simulink model "ThreeDOF_Rocket_Simulator_CD"  (R2023b)
settings: Solver=VariableStepAuto  StartTime=0.0  StopTime=40  FixedStep=1e-4  RelTol=1e-6
libraries: shared3dof x1
settings Model: Creator=giuse  LastModifiedBy=aleco
settings SolverCC: EnableFixedStepZeroCrossing=on
settings DataIOCC: SaveState=on
settings DebuggingCC: UnconnectedInputMsg=warning  UnconnectedOutputMsg=warning  UnconnectedLineMsg=warning
settings ModelReferenceCC: EnableRefExpFcnMdlSchedulingChecks=on
settings RTWCC: DLArmComputeVersion=19.05

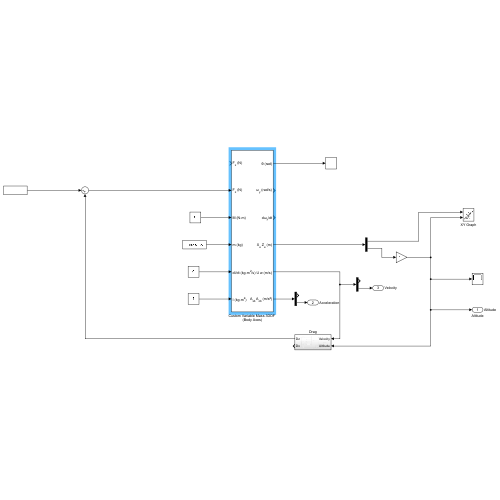
[thumbnail: Simulink's stored preview of the top-level diagram]
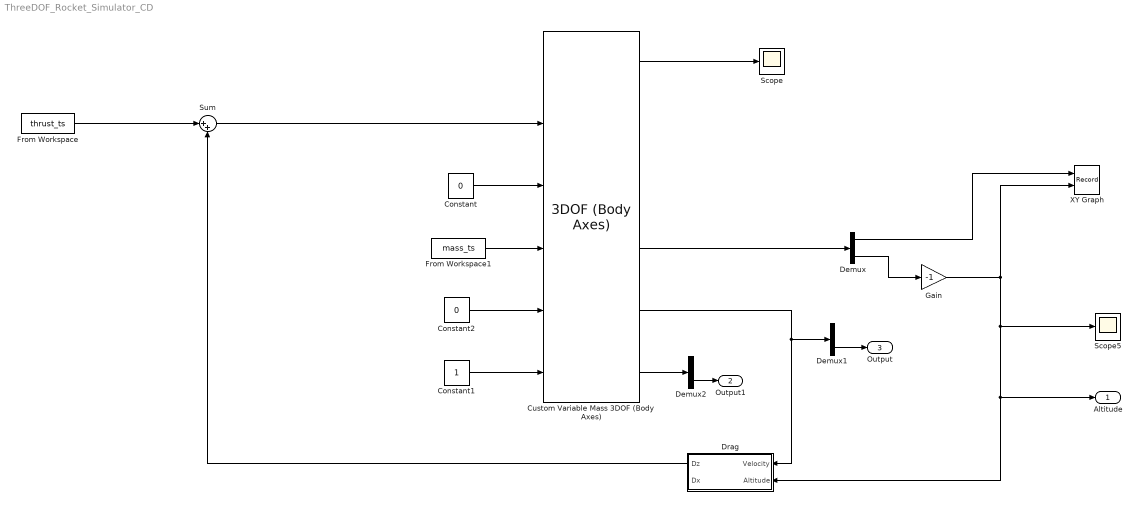
== system ThreeDOF_Rocket_Simulator_CD ==
  Constant : Constant  Value=0
  Constant1 : Constant
  Constant2 : Constant  Value=0
  Custom Variable Mass 3DOF (Body Axes) : shared3dof/3DOF (Body Axes)  units=Metric (MKS)  mtype=Custom Variable  v_ini=0  theta_ini=pi  alpha_ini=0  pos_ini=[0 0]  q_ini=0  mass=1.0  mass_e=0.5  mass_f=3.0  Iyy=1.0  Iyy_e=0.5  Iyy_f=3.0  g_in=Internal  g=9.81  vre_flag=off  abi_flag=off  aMode=0  vel_statename=''  theta_statename=''  pos_statename=''  q_statename=''  mass_statename=''
  Demux : Demux  Outputs=2
  Demux1 : Demux  Outputs=2
  Demux2 : Demux  Outputs=2
  Drag : Subsystem
  From Workspace : FromWorkspace  VariableName=thrust_ts
  From Workspace1 : FromWorkspace  VariableName=mass_ts
  Gain : Gain  Gain=-1
  Scope : Scope
  Scope5 : Scope
  Sum : Sum  Inputs=|++
  XY Graph : Record  FileSettingsInternal="{\"entries\":[{\"content\":{\"excelSettings\":{\"content\":{},\"type\":\"Streamout.ExcelSettings\"}},\"type\":\"Streamout.FileSettingStorage\",\"uuid\":\"\"}],\"packageUris\":[\"http:\\/\\/schema.mathworks.com\\/mf0\\/streamout_blocks\\/R2020a\"],\"version\":\"1.0\"}"  Layout=[1 1]  SignalsInternal="{\"entries\":[{\"content\":{\"signals\":[{\"content\":{\"blockPath\":[],\"dimensions\":[1],\"domain\":\"\",\"lineColor\":\"#a2142f\",\"plots\":[ 1 ],\"port\":1,\"signalID\":1,\"signalName\":\"Demux:1\"},\"type\":\"RecordBlkView.Signal\",\"uuid\":\"\"},{\"content\":{\"blockPath\":[],\"dimensions\":[1],\"domain\":\"\",\"lineColor\":\"#139fff\",\"plots\":[ 1 ],\"port\":2,\"signalID\":2,\"signalName\":\"Gain\"},\"type\":\"RecordBlkView.Signal\",\"uuid\":\"\"}]},\"type\":\"RecordBlkView.InputSignals\",\"uuid\":\"\"}],\"packageUris\":[\"http:\\/\\/schema.mathworks.com\\/mf0\\/streamout_blocks\\/R2020a\"],\"version\":\"1.0\"}"  VisualizationBindings="{\"xyplotplugin\":{\"info\":[{\"series\":[{\"bindingParametersList\":[{\"parameter\":\"X-Axis\",\"signalID\":1,\"signalName\":\"Demux:1\"},{\"parameter\":\"Y-Axis\",\"signalID\":2,\"signalName\":\"Gain\"}],\"seriesID\":0}],\"subplotID\":1}]}}"  CompatibilityTag=XY  st=-1
  Altitude : Outport  SignalName=Altitude
  Output1 : Outport  Port=2  SignalName=Acceleration
  Output : Outport  Port=3  SignalName=Velocity
  wires:
  From Workspace1/1 -> Custom Variable Mass 3DOF (Body Axes)/4
  Gain/1 -> Scope5/1, Altitude/1, Drag/2(Altitude), XY Graph/2
  Demux/2 -> Gain/1
  Demux/1 -> XY Graph/1
  Custom Variable Mass 3DOF (Body Axes)/4 -> Demux/1
  Custom Variable Mass 3DOF (Body Axes)/5 -> Demux1/1, Drag/1(Velocity)
  Drag/1(Dz) -> Sum/2
  From Workspace/1 -> Sum/1
  Sum/1 -> Custom Variable Mass 3DOF (Body Axes)/2
  Custom Variable Mass 3DOF (Body Axes)/1 -> Scope/1
  Constant/1 -> Custom Variable Mass 3DOF (Body Axes)/3
  Constant1/1 -> Custom Variable Mass 3DOF (Body Axes)/6
  Constant2/1 -> Custom Variable Mass 3DOF (Body Axes)/5
  Demux1/2 -> Output/1
  Custom Variable Mass 3DOF (Body Axes)/6 -> Demux2/1
  Demux2/2 -> Output1/1

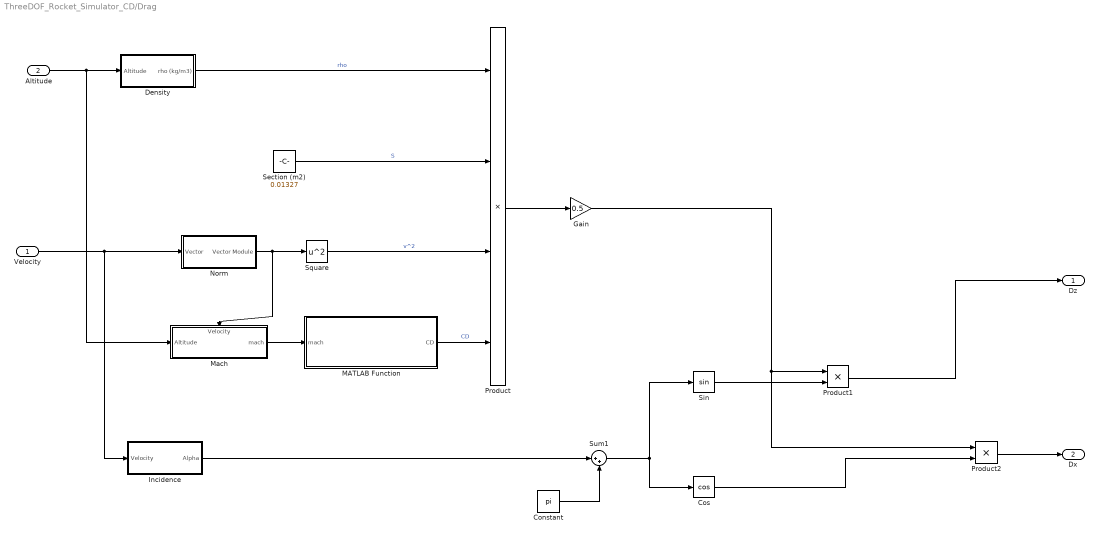
== system ThreeDOF_Rocket_Simulator_CD/Drag ==
  Velocity : Inport
  Altitude : Inport  Port=2
  Constant : Constant  Value=pi
  Cos : Trigonometry  Operator=cos
  Density : Subsystem
  Gain : Gain  Gain=0.5
  Incidence : Subsystem
  MATLAB Function : MATLAB Function  TreatAsAtomicUnit=on
  Mach : Subsystem
      settings: PortSchema="{\"entries\":[{\"content\":{\"sides\":[{\"content\":{\"connectorIds\":[\"In1\"]},\"type\":\"ConnectorPlacement.EquallySpacedRectSide\",\"uuid\":\"3d39723d-d359-4481-8e57-a1560243478f\"},{\"content\":{\"connectorIds\":[\"Out1\"],\"side\":\"RIGHT\"},\"type\":\"ConnectorPlacement.EquallySpacedRectSide\",\"uuid\":\"25d074cf-118b-4153-b466-e753361fe918\"},{\"content\":{\"connectorIds\":[\"In2\"],\"side\":\"TOP\"},\"type\":\"ConnectorPlacement.EquallySpacedRectSide\",\"uuid\":\"b814a212-e79e-4e83-ade8-85d301fd4927\"}]},\"type\":\"ConnectorPlacement.EquallySpacedConnector\",\"uuid\":\"c89f41df-1f7d-46ca-b296-160aff391222\"}],\"packageUris\":[\"http://schema.mathworks.com/mf0/Connector/R2020b\"],\"version\":\"1.0\"}"
  Norm : Subsystem
  Product : Product  Inputs=4
  Product1 : Product
  Product2 : Product
  Section (m2) : Constant  Value=0.01327
  Sin : Trigonometry
  Square : Math  Operator=square
  Sum1 : Sum  Inputs=|++
  Dz : Outport
  Dx : Outport  Port=2
  wires:
  Incidence/1(Alpha) -> Sum1/1
  Norm/1(Vector Module) -> Square/1, Mach/2(Velocity)
  Density/1(rho (kg/m3)) -> Product/1  "rho"
  Section (m2)/1 -> Product/2  "S"
  Square/1 -> Product/3  "v^2"
  Product/1 -> Gain/1
  MATLAB Function/1(CD) -> Product/4  "CD"
  Constant/1 -> Sum1/2
  Sum1/1 -> Sin/1, Cos/1
  Sin/1 -> Product1/2
  Gain/1 -> Product2/1, Product1/1
  Cos/1 -> Product2/2
  Product2/1 -> Dx/1
  Product1/1 -> Dz/1
  Mach/1(mach) -> MATLAB Function/1(mach)
  Altitude/1 -> Mach/1(Altitude), Density/1(Altitude)
  Velocity/1 -> Incidence/1(Velocity), Norm/1(Vector)

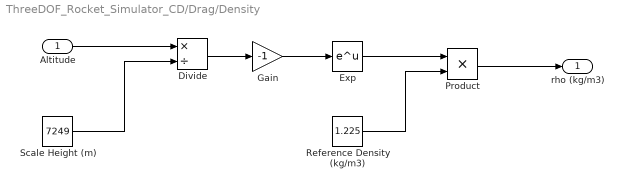
== system ThreeDOF_Rocket_Simulator_CD/Drag/Density ==
  Altitude : Inport
  Divide : Product  Inputs=*/
  Exp : Math
  Gain : Gain  Gain=-1
  Product : Product
  Reference Density (kg/m3) : Constant  Value=1.225
  Scale Height (m) : Constant  Value=7249
  rho (kg/m3) : Outport
  wires:
  Altitude/1 -> Divide/1
  Scale Height (m)/1 -> Divide/2
  Divide/1 -> Gain/1
  Gain/1 -> Exp/1
  Exp/1 -> Product/1
  Reference Density (kg/m3)/1 -> Product/2
  Product/1 -> rho (kg/m3)/1

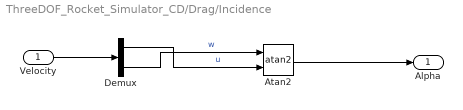
== system ThreeDOF_Rocket_Simulator_CD/Drag/Incidence ==
  Velocity : Inport
  Atan2 : Trigonometry  Operator=atan2
  Demux : Demux  Outputs=2
  Alpha : Outport
  wires:
  Velocity/1 -> Demux/1
  Demux/2 -> Atan2/1  "w"
  Demux/1 -> Atan2/2  "u"
  Atan2/1 -> Alpha/1

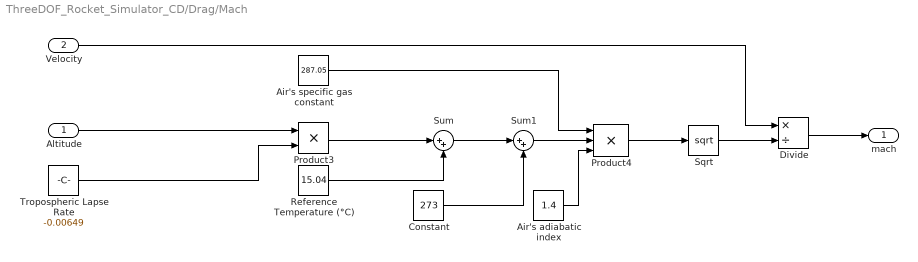
== system ThreeDOF_Rocket_Simulator_CD/Drag/Mach ==
  Altitude : Inport
  Velocity : Inport  Port=2
  Air's adiabatic index : Constant  Value=1.4
  Air's specific gas constant : Constant  Value=287.05
  Constant : Constant  Value=273
  Divide : Product  Inputs=*/
  Product3 : Product
  Product4 : Product  Inputs=3
  Reference Temperature (°C) : Constant  Value=15.04
  Sqrt : Sqrt
  Sum : Sum  Inputs=|++
  Sum1 : Sum  Inputs=|++
  Tropospheric Lapse Rate : Constant  Value=-0.00649
  mach : Outport
  wires:
  Product4/1 -> Sqrt/1
  Product3/1 -> Sum/1
  Air's adiabatic index/1 -> Product4/3
  Tropospheric Lapse Rate/1 -> Product3/2
  Air's specific gas constant/1 -> Product4/1
  Sum/1 -> Sum1/1
  Reference Temperature (°C)/1 -> Sum/2
  Altitude/1 -> Product3/1
  Velocity/1 -> Divide/1
  Divide/1 -> mach/1
  Constant/1 -> Sum1/2
  Sum1/1 -> Product4/2
  Sqrt/1 -> Divide/2

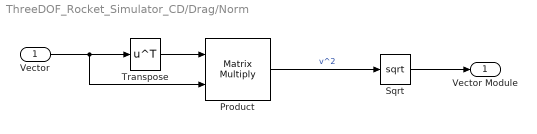
== system ThreeDOF_Rocket_Simulator_CD/Drag/Norm ==
  Vector : Inport
  Product : Product  Multiplication=Matrix(*)
  Sqrt : Sqrt
  Transpose : Math  Operator=transpose
  Vector Module : Outport
  wires:
  Vector/1 -> Product/2, Transpose/1
  Product/1 -> Sqrt/1  "v^2"
  Sqrt/1 -> Vector Module/1
  Transpose/1 -> Product/1

== matlab function ThreeDOF_Rocket_Simulator_CD/Drag/MATLAB Function ==
  data: CD output; mach input
function CD = mach_interp(mach)
cd_table = [0,0
0.01,0.717
0.10,0.509
0.20,0.466
0.30,0.445
0.40,0.442
0.50,0.439
0.60,0.436
0.70,0.440
0.80,0.445
0.90,0.458
1.00,0.556
1.10,0.716
1.20,0.705
1.30,0.668
1.40,0.640
1.50,0.617
1.60,0.597
1.70,0.579
1.80,0.560
1.90,0.545];
CD = spline(cd_table(:,1),cd_table(:,2),mach);
